simulink library "bcm"  (R2021b)
settings: Solver=VariableStepAuto  StartTime=0.0  StopTime=10.0  RelTol=1e-3
undefined symbols (not defined in the file or in its folder): KBCM_BSDFlashOFFT_cnt, KBCM_BSDFlashONT_cnt, KBCM_BSDRedMode_enum, KBCM_BSDWarnReqLv_enum, KBCM_FireBuzzerEN_flg, KBCM_FLTurnLPLv_A, KBCM_FRTurnLPLv_A, KBCM_LampOFFV_V, KBCM_LampONV_V, KBCM_LightDelayOFFT_Cnt, KBCM_LightDelayONT_Cnt, KBCM_RLTurnLPLv_A, KBCM_RRTurnLPLv_A
libraries: simulink x103, hdlsllib x1
(part 2 of 3)

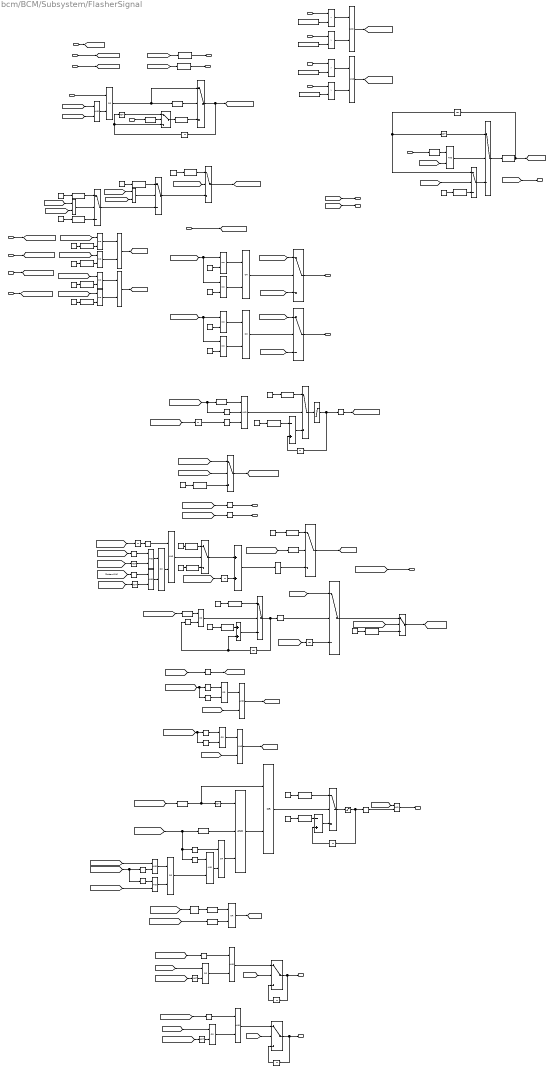
== system bcm/BCM/Subsystem/FlasherSignal ==
  IG1 : Inport
  VINP_LTurnSW_flg : Inport  Port=2
  VINP_RTurnSW_flg : Inport  Port=3
  VINP_VCUHVILSta_flg : Inport  Port=4
  VINP_HazardSW_flg : Inport  Port=5
  VINP_LBSDWarnLv_enum : Inport  Port=6
  VINP_RBSDWarnLv_enum : Inport  Port=7
  VINP_LeftWarnMode_enum : Inport  Port=8
  VINP_RightWarnMode_enum : Inport  Port=9
  PLamp : Inport  Port=10
  VINP_ZFRBCMLFTurnLpCSta_A : Inport  Port=11
  VINP_ZRRBCMLRTurnLpCSta_A : Inport  Port=12
  VINP_ZFRBCMRFTurnLpCSta_A : Inport  Port=13
  VINP_ZRRBCMRRTurnLpCSta_A : Inport  Port=14
  VINP_IVIBuzzerMuteSWSta_flg : Inport  Port=15
  Add : Sum  Inputs=-+
  Add1 : Sum
  Add2 : Sum
  Add3 : Sum  Inputs=-+
  Bit Shift : hdlsllib/Logic and Bit Operations/Bit Shift  mode=Shift Right Logical  N=1
  Bitwise AND : simulink/Logic and Bit Operations/Bitwise Operator  logicop=AND  UseBitMask=on  BitMask=bin2dec('00000011')  BitMaskRealWorld=Stored Integer
  Compare To Constant : simulink/Logic and Bit Operations/Compare To Constant  relop=>  const=0  OutDataTypeStr=boolean
  Compare To Constant1 : simulink/Logic and Bit Operations/Compare To Constant  relop=>  const=0  OutDataTypeStr=boolean
  Compare To Constant10 : simulink/Logic and Bit Operations/Compare To Constant  relop=<  const=2  OutDataTypeStr=boolean
  Compare To Constant11 : simulink/Logic and Bit Operations/Compare To Constant  relop===  const=1  OutDataTypeStr=boolean
  Compare To Constant{3,8,12,17,21} (5 alike) : simulink/Logic and Bit Operations/Compare To Constant  relop===  const=2  OutDataTypeStr=boolean
  Compare To Constant13 : simulink/Logic and Bit Operations/Compare To Constant  relop===  const=1  OutDataTypeStr=boolean
  Compare To Constant{4,9,14,18,23} (5 alike) : simulink/Logic and Bit Operations/Compare To Constant  relop===  const=3  OutDataTypeStr=boolean
  Compare To Constant15 : simulink/Logic and Bit Operations/Compare To Constant  relop===  const=0  OutDataTypeStr=boolean
  Compare To Constant16 : simulink/Logic and Bit Operations/Compare To Constant  relop===  const=1  OutDataTypeStr=boolean
  Compare To Constant19 : simulink/Logic and Bit Operations/Compare To Constant  relop=>  const=0  OutDataTypeStr=boolean
  Compare To Constant2 : simulink/Logic and Bit Operations/Compare To Constant  relop===  const=0  OutDataTypeStr=boolean
  Compare To Constant5 : simulink/Logic and Bit Operations/Compare To Constant  relop=>=  const=17  OutDataTypeStr=boolean
  Compare To Constant6 : simulink/Logic and Bit Operations/Compare To Constant  relop=>=  const=17  OutDataTypeStr=boolean
  Compare To Constant7 : simulink/Logic and Bit Operations/Compare To Constant  relop===  const=0  OutDataTypeStr=boolean
  Constant{,8,10,17..18,20,23,26} (8 alike) : Constant
  Constant{1,4,6,9} (4 alike) : Constant  Value=2
  Constant11 : Constant  Value=3
  Constant12 : Constant  Value=KBCM_FLTurnLPLv_A
  Constant13 : Constant  Value=KBCM_RLTurnLPLv_A
  Constant14 : Constant  Value=KBCM_FRTurnLPLv_A
  Constant15 : Constant  Value=KBCM_RRTurnLPLv_A
  Constant16 : Constant  Value=12
  Constant{3,19,21..22,25} (5 alike) : Constant  Value=0
  Constant2 : Constant  Value=3
  Constant27 : Constant  Value=3
  Constant28 : Constant  Value=10
  Constant5 : Constant  Value=11
  Constant7 : Constant  Value=11
  Data Type Conversion : DataTypeConversion  OutDataTypeStr=boolean
  Data Type Conversion{1..8,12..15,17..19} (15 alike) : DataTypeConversion  OutDataTypeStr=uint8
  Data Type Conversion{9..11,20} (4 alike) : DataTypeConversion  OutDataTypeStr=int8
  Data Type Conversion16 : DataTypeConversion  OutDataTypeStr=boolean
  Data Type Conversion21 : DataTypeConversion  OutDataTypeStr=boolean
  Data Type Conversion22 : DataTypeConversion
  Data Type Conversion23 : DataTypeConversion
  Detect Change{,1..6} (7 alike) : simulink/Logic and Bit Operations/Detect Change  vinit=0  OutDataTypeStr=boolean
  Detect Increase : simulink/Logic and Bit Operations/Detect Increase  vinit=0.0  OutDataTypeStr=boolean
  Detect Increase1 : simulink/Logic and Bit Operations/Detect Increase  vinit=0.0  OutDataTypeStr=boolean
  Detect Increase2 : simulink/Logic and Bit Operations/Detect Increase  vinit=0.0  OutDataTypeStr=boolean
  Logical Operator{,3..6,9..10,17..19,23,25..26,29..30,33,35..36,38} (19 alike) : Logic  AllPortsSameDT=off  OutDataTypeStr=boolean
  Logical Operator{1,13..15,37,39..40} (7 alike) : Logic  Operator=NOT  AllPortsSameDT=off  OutDataTypeStr=boolean
  Logical Operator11 : Logic  Inputs=3  AllPortsSameDT=off  OutDataTypeStr=boolean
  Logical Operator{2,7..8,12,20..22,24,27..28,31..32,34} (13 alike) : Logic  Operator=OR  AllPortsSameDT=off  OutDataTypeStr=boolean
  Logical Operator16 : Logic  Inputs=3  AllPortsSameDT=off  OutDataTypeStr=boolean
  Relational Operator{,1..7} (8 alike) : RelationalOperator  Operator===  OutDataTypeStr=boolean  RndMeth=Simplest
  Relational Operator{8..11} (4 alike) : RelationalOperator  Operator=>  OutDataTypeStr=boolean  RndMeth=Simplest
  Saturation : Saturate  UpperLimit=12  LowerLimit=0
  Saturation1 : Saturate  UpperLimit=10  LowerLimit=0
  Switch{,1..18} (19 alike) : Switch  Criteria=u2 > Threshold
  Unit Delay{,1..10} (11 alike) : UnitDelay  SampleTime=-1  HasFrameUpgradeWarning=on
  VBCM_FDCBCMSMKLCmd_flg : Outport
  VBCM_FDCBCMSMKRCmd_flg : Outport  Port=2
  VBCM_FDCBCMDVRSignalLCmd_flg : Outport  Port=3
  VBCM_FDCBCMDVRSignalRCmd_flg : Outport  Port=4
  VBCM_FDCBCMBSDBuzzerCmd_flg : Outport  Port=5
  VBCM_FDCBCMSLTLpCmd_flg : Outport  Port=6
  VBCM_FDCBCMSRTLpCmd_flg : Outport  Port=7
  VBCM_FDCBCMLTurnLpCmd_flg : Outport  Port=8
  VBCM_FDCBCMRTurnLpCmd_flg : Outport  Port=9
  PatternOld : Outport  Port=10
  VBCM_FDCBCMLTurnSWSta_flg : Outport  Port=11
  VBCM_FDCBCMRTurnSWSta_flg : Outport  Port=12
  VBCM_FDCBCMTurnBuzzerENSta_flg : Outport  Port=13
  wires:
  VINP_HazardSW_flg/1 -> Detect Increase/1
  Unit Delay/1 -> Switch/3, Logical Operator1/1
  Switch/1 -> Data Type Conversion/1
  Data Type Conversion/1 -> Switch1/3
  Detect Increase/1 -> Switch/2
  Logical Operator1/1 -> Switch/1
  VINP_LTurnSW_flg/1 -> [VINP_LTurnSW_flg]
  VINP_RTurnSW_flg/1 -> [VINP_RTurnSW_flg]
  [VINP_LTurnSW_flg] -> Logical Operator/1
  [VINP_RTurnSW_flg] -> Logical Operator/2
  Logical Operator2/1 -> Detect Change6/1, Switch1/1
  Switch1/1 -> Unit Delay/1, [HazardSW]
  Logical Operator/1 -> Logical Operator2/2
  VINP_VCUHVILSta_flg/1 -> Logical Operator2/1
  Switch2/1 -> Switch3/3
  Switch3/1 -> Switch4/3
  [HazardSW] -> Switch4/2
  Data Type Conversion1/1 -> Switch4/1
  Constant/1 -> Data Type Conversion1/1
  IG1/1 -> [IG1]
  Logical Operator3/1 -> Switch3/2
  [IG1] -> Logical Operator3/1
  [VINP_LTurnSW_flg] -> Logical Operator3/2
  Constant1/1 -> Data Type Conversion2/1
  Data Type Conversion2/1 -> Switch3/1
  Data Type Conversion3/1 -> Switch2/1
  Constant2/1 -> Data Type Conversion3/1
  [VINP_RTurnSW_flg] -> Logical Operator4/2
  [IG1] -> Logical Operator4/1
  Logical Operator4/1 -> Switch2/2
  Constant3/1 -> Data Type Conversion4/1
  Data Type Conversion4/1 -> Switch2/3
  Switch4/1 -> [PatternNew]
  Constant4/1 -> Data Type Conversion5/1
  Data Type Conversion5/1 -> Relational Operator/2
  Data Type Conversion6/1 -> Relational Operator1/2
  Constant5/1 -> Data Type Conversion6/1
  Relational Operator/1 -> Logical Operator5/1
  Relational Operator1/1 -> Logical Operator5/2
  Logical Operator5/1 -> [LBSD_En]
  Logical Operator6/1 -> [RBSD_En]
  Relational Operator3/1 -> Logical Operator6/2
  Relational Operator2/1 -> Logical Operator6/1
  Constant7/1 -> Data Type Conversion8/1
  Data Type Conversion8/1 -> Relational Operator3/2
  Data Type Conversion7/1 -> Relational Operator2/2
  Constant6/1 -> Data Type Conversion7/1
  [PatternOld] -> Relational Operator5/1, Relational Operator4/1
  Constant8/1 -> Relational Operator4/2
  Constant9/1 -> Relational Operator5/2
  PLamp/1 -> [PLamp]
  Relational Operator4/1 -> Logical Operator7/1
  Relational Operator5/1 -> Logical Operator7/2
  Logical Operator7/1 -> Switch5/2
  [PLamp] -> Switch5/3
  [LTurnLP] -> Switch5/1
  Switch5/1 -> VBCM_FDCBCMSMKLCmd_flg/1
  Switch6/1 -> VBCM_FDCBCMSMKRCmd_flg/1
  [RTurnLP] -> Switch6/1
  [PLamp] -> Switch6/3
  Logical Operator8/1 -> Switch6/2
  Relational Operator7/1 -> Logical Operator8/2
  Relational Operator6/1 -> Logical Operator8/1
  Constant11/1 -> Relational Operator7/2
  Constant10/1 -> Relational Operator6/2
  [PatternOld] -> Relational Operator6/1, Relational Operator7/1
  VINP_ZFRBCMLFTurnLpCSta_A/1 -> Relational Operator8/1
  Constant12/1 -> Relational Operator8/2
  VINP_ZRRBCMLRTurnLpCSta_A/1 -> Relational Operator9/1
  Constant13/1 -> Relational Operator9/2
  VINP_ZFRBCMRFTurnLpCSta_A/1 -> Relational Operator10/1
  Constant14/1 -> Relational Operator10/2
  Constant15/1 -> Relational Operator11/2
  VINP_ZRRBCMRRTurnLpCSta_A/1 -> Relational Operator11/1
  Relational Operator8/1 -> Logical Operator9/1
  Relational Operator9/1 -> Logical Operator9/2
  Logical Operator9/1 -> [LTurnLPOK]
  Relational Operator10/1 -> Logical Operator10/1
  Relational Operator11/1 -> Logical Operator10/2
  Logical Operator10/1 -> [RTurnLPOK]
  [LTurnLP] -> VBCM_FDCBCMLTurnLpCmd_flg/1
  [RTurnLP] -> VBCM_FDCBCMRTurnLpCmd_flg/1
  [PatternOld] -> Detect Change4/1
  Compare To Constant17/1 -> Logical Operator18/2
  Add3/1 -> Switch13/3
  [LampON] -> Logical Operator28/1
  [RBSD_En] -> Logical Operator40/1
  [LBSD_En] -> Logical Operator39/1
  Saturation1/1 -> Compare To Constant19/1, Unit Delay7/1
  [LTurnLPOK] -> Logical Operator13/1
  [STurnUpdate] -> Switch15/2
  Detect Change4/1 -> Logical Operator24/2
  Bit Shift/1 -> Detect Change5/1
  [Step] -> Bit Shift/1
  Compare To Constant15/1 -> Logical Operator21/1
  [PatternOld] -> Detect Increase1/1
  [LampON] -> Logical Operator27/1
  Switch16/1 -> Unit Delay9/1, VBCM_FDCBCMSRTLpCmd_flg/1
  [LBSD_En] -> Logical Operator18/1
  [PatternOld] -> Compare To Constant18/1, Compare To Constant17/1
  Logical Operator16/1 -> Logical Operator22/2
  Switch10/1 -> Switch14/1
  Compare To Constant19/1 -> Logical Operator38/2
  Compare To Constant23/1 -> Logical Operator26/1
  Add2/1 -> Bitwise AND/1
  [Step] -> Unit Delay6/1
  Unit Delay8/1 -> Switch15/3
  Logical Operator24/1 -> [STurnUpdate]
  Detect Change3/1 -> Logical Operator16/2
  Constant18/1 -> Data Type Conversion11/1
  Detect Change5/1 -> Logical Operator24/1
  Switch13/1 -> Saturation1/1
  Logical Operator20/1 -> Logical Operator17/2
  Detect Increase1/1 -> Logical Operator22/1, Logical Operator15/1
  Logical Operator15/1 -> Logical Operator16/1
  Compare To Constant18/1 -> Logical Operator19/1
  Logical Operator22/1 -> Switch13/2
  Unit Delay9/1 -> Switch16/3
  [RBSD_En] -> Logical Operator19/2
  Logical Operator27/1 -> Logical Operator25/2
  [PatternOld] -> Compare To Constant21/1
  [PatternOld] -> Compare To Constant23/1
  [PatternOld] -> Switch14/2
  Logical Operator25/1 -> Switch15/1
  Constant19/1 -> Data Type Conversion12/1
  Switch12/1 -> Add2/1
  Logical Operator19/1 -> Logical Operator20/2
  Switch14/1 -> [Step]
  Compare To Constant11/1 -> Logical Operator32/1
  Logical Operator32/1 -> Logical Operator33/1
  [NextStep] -> Switch10/1
  Logical Operator14/1 -> Logical Operator30/2
  Unit Delay4/1 -> Compare To Constant7/1
  Compare To Constant10/1 -> [LampON]
  [Step] -> Compare To Constant10/1
  Data Type Conversion12/1 -> Switch14/3
  Data Type Conversion11/1 -> Add3/1
  Compare To Constant12/1 -> Logical Operator32/2
  Constant28/1 -> Data Type Conversion20/1
  [RTurnLPOK] -> Logical Operator14/1
  [LampON] -> Logical Operator35/2
  Compare To Constant14/1 -> Logical Operator34/2
  Compare To Constant16/1 -> Logical Operator17/1
  Logical Operator34/1 -> Logical Operator35/1
  Data Type Conversion19/1 -> Switch12/1
  [Step] -> Unit Delay4/1
  Constant27/1 -> Data Type Conversion19/1
  Logical Operator29/1 -> Logical Operator31/1
  [PatternOld] -> Unit Delay2/1
  Data Type Conversion15/1 -> Add1/1
  Constant23/1 -> Data Type Conversion15/1
  [Step] -> Unit Delay5/1
  [Step] -> Detect Change3/1, Compare To Constant15/1, Compare To Constant16/1
  Logical Operator17/1 -> Logical Operator21/2
  Data Type Conversion18/1 -> Switch12/3
  Unit Delay3/1 -> Compare To Constant5/1, Add1/2
  [PatternOld] -> Compare To Constant3/1
  Bitwise AND/1 -> Switch11/3
  Logical Operator31/1 -> Logical Operator23/2
  Logical Operator11/1 -> Switch7/2
  Add/1 -> Switch7/3
  Compare To Constant6/1 -> Switch10/2
  Constant16/1 -> Data Type Conversion9/1
  Add1/1 -> Switch9/3
  [PatternOld] -> Compare To Constant4/1
  Compare To Constant/1 -> Logical Operator11/3
  Detect Change/1 -> Logical Operator11/1
  Logical Operator30/1 -> Logical Operator31/2
  Unit Delay1/1 -> Add/2
  Logical Operator26/1 -> Switch16/1
  Unit Delay5/1 -> Switch10/3
  Compare To Constant5/1 -> Logical Operator12/2
  [SwitchAllow] -> Switch8/2
  [LampON] -> Logical Operator33/2
  [PatternOld] -> Compare To Constant8/1
  [PatternNew] -> Detect Change/1, Compare To Constant1/1
  Constant25/1 -> Data Type Conversion17/1
  Unit Delay7/1 -> Add3/2
  Constant17/1 -> Data Type Conversion10/1
  Logical Operator28/1 -> Logical Operator26/2
  [STurnUpdate] -> Switch16/2
  Compare To Constant8/1 -> Logical Operator29/1
  Compare To Constant7/1 -> Logical Operator23/1
  Constant22/1 -> Data Type Conversion14/1
  Compare To Constant9/1 -> Logical Operator30/1
  Unit Delay2/1 -> Compare To Constant/1
  Data Type Conversion10/1 -> Add/1
  Switch15/1 -> Unit Delay8/1, VBCM_FDCBCMSLTLpCmd_flg/1
  Detect Change1/1 -> Logical Operator12/1
  Compare To Constant21/1 -> Logical Operator25/1
  Data Type Conversion9/1 -> Switch7/1
  Logical Operator12/1 -> Switch9/2
  Switch11/1 -> [NextStep]
  Switch7/1 -> Saturation/1
  [PatternOld] -> Compare To Constant9/1
  Unit Delay6/1 -> Add2/2
  Logical Operator21/1 -> Logical Operator16/3
  Logical Operator18/1 -> Logical Operator20/1
  Data Type Conversion14/1 -> Switch9/1
  Detect Change2/1 -> Switch11/2
  [PatternOld] -> Detect Change1/1
  Data Type Conversion13/1 -> Switch8/3
  Constant21/1 -> Data Type Conversion13/1
  [PatternOld] -> Compare To Constant13/1, Compare To Constant14/1
  Compare To Constant3/1 -> VBCM_FDCBCMDVRSignalLCmd_flg/1
  Constant26/1 -> Data Type Conversion18/1
  Compare To Constant2/1 -> [SwitchAllow]
  [PatternOld] -> Detect Change2/1
  Data Type Conversion20/1 -> Switch13/1
  Compare To Constant4/1 -> VBCM_FDCBCMDVRSignalRCmd_flg/1
  Switch8/1 -> [PatternOld]
  Compare To Constant13/1 -> Logical Operator34/1
  Logical Operator13/1 -> Logical Operator29/2
  [PatternNew] -> Switch8/1
  [PatternOld] -> Compare To Constant12/1, Compare To Constant11/1
  Compare To Constant1/1 -> Logical Operator11/2
  Logical Operator23/1 -> Switch12/2
  Switch9/1 -> Compare To Constant6/1, Unit Delay3/1
  Data Type Conversion17/1 -> Switch11/1
  Saturation/1 -> Unit Delay1/1, Compare To Constant2/1
  Logical Operator33/1 -> [LTurnLP]
  Logical Operator35/1 -> [RTurnLP]
  [PatternOld] -> PatternOld/1
  VINP_LBSDWarnLv_enum/1 -> [VINP_LBSDWarnLv_enum]
  [VINP_LBSDWarnLv_enum] -> Relational Operator/1
  VINP_LeftWarnMode_enum/1 -> [VINP_LeftWarnMode_enum]
  [VINP_LeftWarnMode_enum] -> Relational Operator1/1
  VINP_RBSDWarnLv_enum/1 -> [VINP_RBSDWarnLv_enum]
  [VINP_RBSDWarnLv_enum] -> Relational Operator2/1
  VINP_RightWarnMode_enum/1 -> [VINP_RightWarnMode_enum]
  [VINP_RightWarnMode_enum] -> Relational Operator3/1
  Detect Change6/1 -> Switch1/2
  [VINP_LTurnSW_flg] -> Data Type Conversion22/1
  [VINP_RTurnSW_flg] -> Data Type Conversion23/1
  VINP_IVIBuzzerMuteSWSta_flg/1 -> Detect Increase2/1
  Detect Increase2/1 -> Logical Operator36/1
  [IG1] -> Logical Operator36/2
  Logical Operator36/1 -> Switch17/2
  Logical Operator37/1 -> Switch17/1
  Switch17/1 -> Data Type Conversion16/1
  Data Type Conversion16/1 -> [TurnBuzzerEN], Unit Delay10/1
  Switch18/1 -> Switch17/3
  [IG1] -> Switch18/2
  Data Type Conversion21/1 -> Switch18/3
  Constant20/1 -> Data Type Conversion21/1
  [TurnBuzzerEN] -> VBCM_FDCBCMTurnBuzzerENSta_flg/1
  [TurnBuzzerEN] -> Logical Operator38/1
  Logical Operator38/1 -> VBCM_FDCBCMBSDBuzzerCmd_flg/1
  Logical Operator39/1 -> Logical Operator27/2
  Logical Operator40/1 -> Logical Operator28/2
  Unit Delay10/1 -> Switch18/1, Logical Operator37/1
  Data Type Conversion22/1 -> VBCM_FDCBCMLTurnSWSta_flg/1
  Data Type Conversion23/1 -> VBCM_FDCBCMRTurnSWSta_flg/1

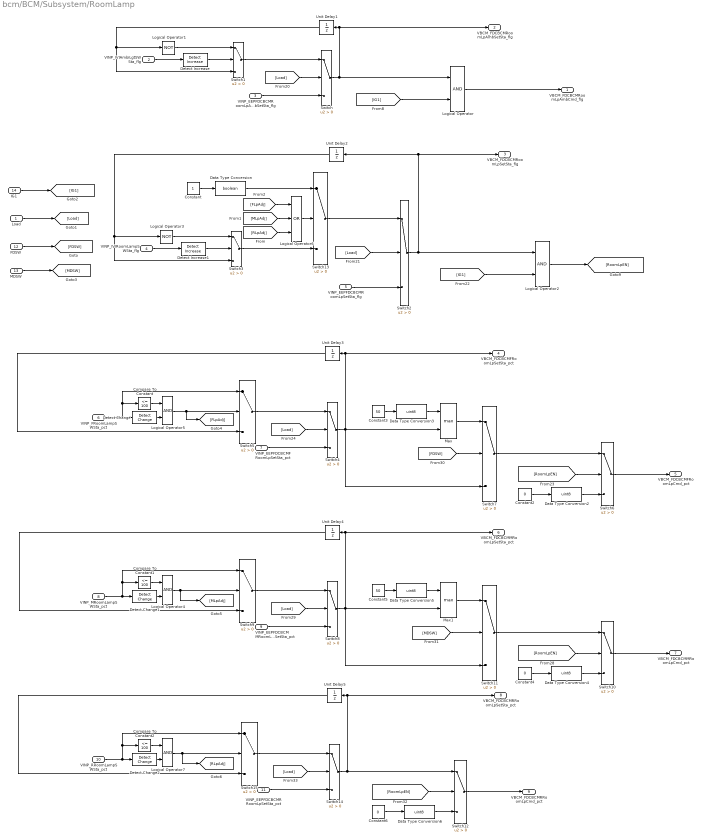
== system bcm/BCM/Subsystem/RoomLamp ==
  Load : Inport
  VINP_IVIAmbiLgtSWSta_flg : Inport  Port=2
  VINP_EEPFDCBCMRoomLpAmbSetSta_flg : Inport  Port=3
  VINP_IVIRoomLampSWSta_flg : Inport  Port=4
  VINP_EEPFDCBCMRoomLpSetSta_flg : Inport  Port=5
  VINP_FRoomLampSWSta_pct : Inport  Port=6
  VINP_EEPFDCBCMFRoomLpSetSta_pct : Inport  Port=7
  VINP_MRoomLampSWSta_pct : Inport  Port=8
  VINP_EEPFDCBCMMRoomLpSetSta_pct : Inport  Port=9
  VINP_RRoomLampSWSta_pct : Inport  Port=10
  VINP_EEPFDCBCMRRoomLpSetSta_pct : Inport  Port=11
  FDSW : Inport  Port=12
  MDSW : Inport  Port=13
  IG1 : Inport  Port=14
  Compare To Constant : simulink/Logic and Bit Operations/Compare To Constant  relop=<=  const=100  OutDataTypeStr=boolean
  Compare To Constant1 : simulink/Logic and Bit Operations/Compare To Constant  relop=<=  const=100  OutDataTypeStr=boolean
  Compare To Constant2 : simulink/Logic and Bit Operations/Compare To Constant  relop=<=  const=100  OutDataTypeStr=boolean
  Constant : Constant
  Constant2 : Constant  Value=0
  Constant3 : Constant  Value=50
  Constant4 : Constant  Value=0
  Constant5 : Constant  Value=50
  Constant6 : Constant  Value=0
  Data Type Conversion : DataTypeConversion  OutDataTypeStr=boolean
  Data Type Conversion{2..6} (5 alike) : DataTypeConversion  OutDataTypeStr=uint8
  Detect Change : simulink/Logic and Bit Operations/Detect Change  vinit=0  OutDataTypeStr=boolean
  Detect Change1 : simulink/Logic and Bit Operations/Detect Change  vinit=0  OutDataTypeStr=boolean
  Detect Change2 : simulink/Logic and Bit Operations/Detect Change  vinit=0  OutDataTypeStr=boolean
  Detect Increase : simulink/Logic and Bit Operations/Detect Increase  vinit=0.0  OutDataTypeStr=boolean
  Detect Increase1 : simulink/Logic and Bit Operations/Detect Increase  vinit=0.0  OutDataTypeStr=boolean
  Logical Operator{,2,4..5,7} (5 alike) : Logic  AllPortsSameDT=off  OutDataTypeStr=boolean
  Logical Operator1 : Logic  Operator=NOT  AllPortsSameDT=off  OutDataTypeStr=boolean
  Logical Operator3 : Logic  Operator=NOT  AllPortsSameDT=off  OutDataTypeStr=boolean
  Logical Operator6 : Logic  Operator=OR  Inputs=3  AllPortsSameDT=off  OutDataTypeStr=boolean
  Max : MinMax  Function=max  Inputs=2
  Max1 : MinMax  Function=max  Inputs=2
  Switch{,1..15} (16 alike) : Switch  Criteria=u2 > Threshold
  Unit Delay{1..5} (5 alike) : UnitDelay  SampleTime=-1  HasFrameUpgradeWarning=on
  VBCM_FDCBCMRoomLpAmbCmd_flg : Outport
  VBCM_FDCBCMRoomLpAmbSetSta_flg : Outport  Port=2
  VBCM_FDCBCMRoomLpSetSta_flg : Outport  Port=3
  VBCM_FDCBCMFRoomLpSetSta_pct : Outport  Port=4
  VBCM_FDCBCMFRoomLpCmd_pct : Outport  Port=5
  VBCM_FDCBCMMRoomLpSetSta_pct : Outport  Port=6
  VBCM_FDCBCMMRoomLpCmd_pct : Outport  Port=7
  VBCM_FDCBCMRRoomLpSetSta_pct : Outport  Port=8
  VBCM_FDCBCMRRoomLpCmd_pct : Outport  Port=9
  wires:
  Data Type Conversion5/1 -> Max1/1
  Logical Operator2/1 -> [RoomLpEN]
  VINP_EEPFDCBCMRRoomLpSetSta_pct/1 -> Switch14/3
  Logical Operator/1 -> VBCM_FDCBCMRoomLpAmbCmd_flg/1
  Compare To Constant/1 -> Logical Operator5/1
  Switch12/1 -> VBCM_FDCBCMRRoomLpCmd_pct/1
  Data Type Conversion2/1 -> Switch6/3
  Switch/1 -> Logical Operator/1, VBCM_FDCBCMRoomLpAmbSetSta_flg/1, Unit Delay1/1
  Logical Operator4/1 -> [MLpAdj], Switch9/2
  VINP_RRoomLampSWSta_pct/1 -> Switch15/1, Compare To Constant2/1, Detect Change2/1
  Switch5/1 -> Switch4/1
  Switch1/1 -> Switch/1
  Switch6/1 -> VBCM_FDCBCMFRoomLpCmd_pct/1
  [FDSW] -> Switch7/2
  Switch14/1 -> Switch12/1, VBCM_FDCBCMRRoomLpSetSta_pct/1, Unit Delay5/1
  [IG1] -> Logical Operator/2
  Switch3/1 -> Switch13/3
  VINP_IVIAmbiLgtSWSta_flg/1 -> Detect Increase/1
  Max1/1 -> Switch11/1
  VINP_IVIRoomLampSWSta_flg/1 -> Detect Increase1/1
  Detect Increase/1 -> Switch1/2
  Unit Delay1/1 -> Logical Operator1/1, Switch1/3
  Data Type Conversion4/1 -> Switch10/3
  [Load] -> Switch2/2
  [MDSW] -> Switch11/2
  Unit Delay2/1 -> Switch3/3, Logical Operator3/1
  Switch2/1 -> Logical Operator2/1, Unit Delay2/1, VBCM_FDCBCMRoomLpSetSta_flg/1
  Logical Operator1/1 -> Switch1/1
  [RoomLpEN] -> Switch6/2
  Logical Operator7/1 -> [RLpAdj], Switch15/2
  VINP_FRoomLampSWSta_pct/1 -> Switch5/1, Compare To Constant/1, Detect Change/1
  Compare To Constant1/1 -> Logical Operator4/1
  Detect Change2/1 -> Logical Operator7/2
  Constant6/1 -> Data Type Conversion6/1
  Constant4/1 -> Data Type Conversion4/1
  [Load] -> Switch/2
  [Load] -> Switch14/2
  Constant3/1 -> Data Type Conversion3/1
  Switch15/1 -> Switch14/1
  VINP_EEPFDCBCMRoomLpAmbSetSta_flg/1 -> Switch/3
  Logical Operator3/1 -> Switch3/1
  Switch7/1 -> Switch6/1
  [IG1] -> Logical Operator2/2
  Switch4/1 -> Switch7/3, VBCM_FDCBCMFRoomLpSetSta_pct/1, Unit Delay3/1, Max/2
  Unit Delay5/1 -> Switch15/3
  Logical Operator5/1 -> [FLpAdj], Switch5/2
  VINP_EEPFDCBCMRoomLpSetSta_flg/1 -> Switch2/3
  Detect Increase1/1 -> Switch3/2
  Data Type Conversion3/1 -> Max/1
  [RoomLpEN] -> Switch12/2
  Data Type Conversion6/1 -> Switch12/3
  Compare To Constant2/1 -> Logical Operator7/1
  [Load] -> Switch4/2
  VINP_EEPFDCBCMFRoomLpSetSta_pct/1 -> Switch4/3
  Unit Delay3/1 -> Switch5/3
  Max/1 -> Switch7/1
  Switch9/1 -> Switch8/1
  Switch11/1 -> Switch10/1
  Constant5/1 -> Data Type Conversion5/1
  Switch10/1 -> VBCM_FDCBCMMRoomLpCmd_pct/1
  Detect Change1/1 -> Logical Operator4/2
  [RoomLpEN] -> Switch10/2
  VINP_MRoomLampSWSta_pct/1 -> Detect Change1/1, Compare To Constant1/1, Switch9/1
  Unit Delay4/1 -> Switch9/3
  Switch8/1 -> Max1/2, VBCM_FDCBCMMRoomLpSetSta_pct/1, Unit Delay4/1, Switch11/3
  Constant2/1 -> Data Type Conversion2/1
  VINP_EEPFDCBCMMRoomLpSetSta_pct/1 -> Switch8/3
  [Load] -> Switch8/2
  Detect Change/1 -> Logical Operator5/2
  FDSW/1 -> [FDSW]
  Load/1 -> [Load]
  IG1/1 -> [IG1]
  MDSW/1 -> [MDSW]
  Switch13/1 -> Switch2/1
  Logical Operator6/1 -> Switch13/2
  [RLpAdj] -> Logical Operator6/3
  [MLpAdj] -> Logical Operator6/2
  [FLpAdj] -> Logical Operator6/1
  Constant/1 -> Data Type Conversion/1
  Data Type Conversion/1 -> Switch13/1

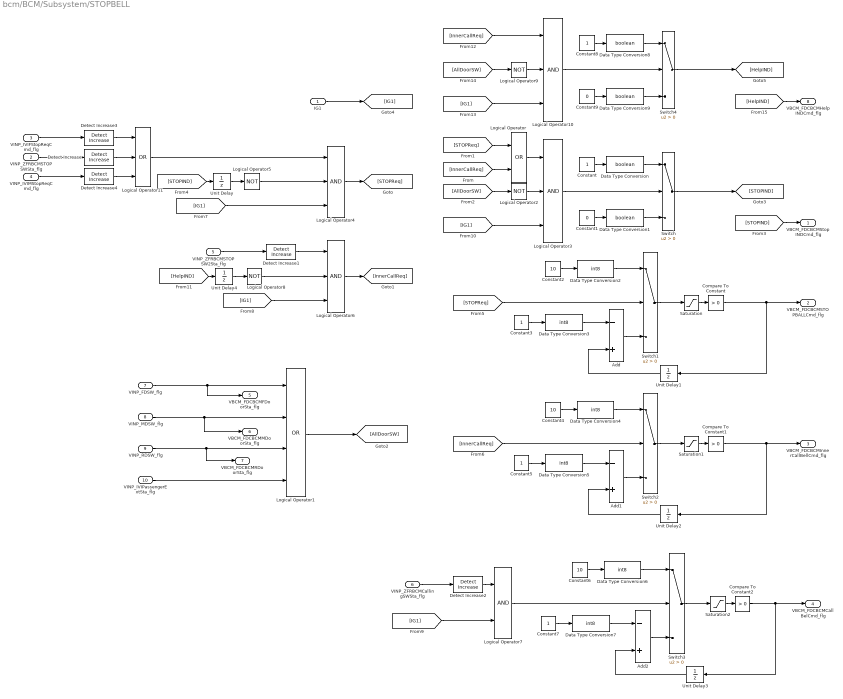
== system bcm/BCM/Subsystem/STOPBELL ==
  IG1 : Inport
  VINP_ZFRBCMSTOPSWSta_flg : Inport  Port=2
  VINP_IVIFStopReqCmd_flg : Inport  Port=3
  VINP_IVIMStopReqCmd_flg : Inport  Port=4
  VINP_ZFRBCMSTOPSW2Sta_flg : Inport  Port=5
  VINP_ZFRBCMCallingSWSta_flg : Inport  Port=6
  VINP_FDSW_flg : Inport  Port=7
  VINP_MDSW_flg : Inport  Port=8
  VINP_RDSW_flg : Inport  Port=9
  VINP_IVIPassengerExtSta_flg : Inport  Port=10
  Add : Sum  Inputs=-+
  Add1 : Sum  Inputs=-+
  Add2 : Sum  Inputs=-+
  Compare To Constant : simulink/Logic and Bit Operations/Compare To Constant  relop=>  const=0  OutDataTypeStr=boolean
  Compare To Constant1 : simulink/Logic and Bit Operations/Compare To Constant  relop=>  const=0  OutDataTypeStr=boolean
  Compare To Constant2 : simulink/Logic and Bit Operations/Compare To Constant  relop=>  const=0  OutDataTypeStr=boolean
  Constant{,3,5,7..8} (5 alike) : Constant
  Constant1 : Constant  Value=0
  Constant2 : Constant  Value=10
  Constant4 : Constant  Value=10
  Constant6 : Constant  Value=10
  Constant9 : Constant  Value=0
  Data Type Conversion{,1,8..9} (4 alike) : DataTypeConversion  OutDataTypeStr=boolean
  Data Type Conversion{2..7} (6 alike) : DataTypeConversion  OutDataTypeStr=int8
  Detect Increase{,1..4} (5 alike) : simulink/Logic and Bit Operations/Detect Increase  vinit=0.0  OutDataTypeStr=boolean
  Logical Operator : Logic  Operator=OR  AllPortsSameDT=off  OutDataTypeStr=boolean
  Logical Operator1 : Logic  Operator=OR  Inputs=4  AllPortsSameDT=off  OutDataTypeStr=boolean
  Logical Operator{3..4,6,10} (4 alike) : Logic  Inputs=3  AllPortsSameDT=off  OutDataTypeStr=boolean
  Logical Operator11 : Logic  Operator=OR  Inputs=3  AllPortsSameDT=off  OutDataTypeStr=boolean
  Logical Operator{2,5,8..9} (4 alike) : Logic  Operator=NOT  AllPortsSameDT=off  OutDataTypeStr=boolean
  Logical Operator7 : Logic  AllPortsSameDT=off  OutDataTypeStr=boolean
  Saturation : Saturate  UpperLimit=10  LowerLimit=0
  Saturation1 : Saturate  UpperLimit=10  LowerLimit=0
  Saturation2 : Saturate  UpperLimit=10  LowerLimit=0
  Switch{,1..4} (5 alike) : Switch  Criteria=u2 > Threshold
  Unit Delay{,1..4} (5 alike) : UnitDelay  SampleTime=-1  HasFrameUpgradeWarning=on
  VBCM_FDCBCMStopINDCmd_flg : Outport
  VBCM_FDCBCMSTOPBALLCmd_flg : Outport  Port=2
  VBCM_FDCBCMInnerCallBellCmd_flg : Outport  Port=3
  VBCM_FDCBCMCallBelCmd_flg : Outport  Port=4
  VBCM_FDCBCMFDoorSta_flg : Outport  Port=5
  VBCM_FDCBCMMDoorSta_flg : Outport  Port=6
  VBCM_FDCBCMRDoorSta_flg : Outport  Port=7
  VBCM_FDCBCMHelpINDCmd_flg : Outport  Port=8
  wires:
  VINP_ZFRBCMSTOPSWSta_flg/1 -> Detect Increase/1
  VINP_ZFRBCMSTOPSW2Sta_flg/1 -> Detect Increase1/1
  [STOPReq] -> Logical Operator/1
  [InnerCallReq] -> Logical Operator/2
  Logical Operator/1 -> Logical Operator3/1
  Constant/1 -> Data Type Conversion/1
  Data Type Conversion/1 -> Switch/1
  VINP_MDSW_flg/1 -> VBCM_FDCBCMMDoorSta_flg/1, Logical Operator1/2
  VINP_FDSW_flg/1 -> VBCM_FDCBCMFDoorSta_flg/1, Logical Operator1/1
  VINP_RDSW_flg/1 -> VBCM_FDCBCMRDoorSta_flg/1, Logical Operator1/3
  Logical Operator1/1 -> [AllDoorSW]
  VINP_IVIPassengerExtSta_flg/1 -> Logical Operator1/4
  [AllDoorSW] -> Logical Operator2/1
  Logical Operator2/1 -> Logical Operator3/2
  Logical Operator3/1 -> Switch/2
  Constant1/1 -> Data Type Conversion1/1
  Data Type Conversion1/1 -> Switch/3
  [STOPIND] -> VBCM_FDCBCMStopINDCmd_flg/1
  Switch/1 -> [STOPIND]
  [STOPIND] -> Unit Delay/1
  VINP_ZFRBCMCallingSWSta_flg/1 -> Detect Increase2/1
  Detect Increase/1 -> Logical Operator11/2
  Unit Delay/1 -> Logical Operator5/1
  Logical Operator4/1 -> [STOPReq]
  Logical Operator5/1 -> Logical Operator4/2
  [STOPReq] -> Switch1/2
  Constant2/1 -> Data Type Conversion2/1
  Data Type Conversion2/1 -> Switch1/1
  Add/1 -> Switch1/3
  Data Type Conversion3/1 -> Add/1
  Constant3/1 -> Data Type Conversion3/1
  Switch1/1 -> Saturation/1
  Saturation/1 -> Compare To Constant/1
  Unit Delay1/1 -> Add/2
  Compare To Constant/1 -> VBCM_FDCBCMSTOPBALLCmd_flg/1, Unit Delay1/1
  Compare To Constant1/1 -> VBCM_FDCBCMInnerCallBellCmd_flg/1, Unit Delay2/1
  Unit Delay2/1 -> Add1/2
  Saturation1/1 -> Compare To Constant1/1
  Switch2/1 -> Saturation1/1
  Constant5/1 -> Data Type Conversion5/1
  Data Type Conversion5/1 -> Add1/1
  Add1/1 -> Switch2/3
  Data Type Conversion4/1 -> Switch2/1
  Constant4/1 -> Data Type Conversion4/1
  [InnerCallReq] -> Switch2/2
  Logical Operator7/1 -> Switch3/2
  Constant6/1 -> Data Type Conversion6/1
  Data Type Conversion6/1 -> Switch3/1
  Add2/1 -> Switch3/3
  Data Type Conversion7/1 -> Add2/1
  Constant7/1 -> Data Type Conversion7/1
  Switch3/1 -> Saturation2/1
  Saturation2/1 -> Compare To Constant2/1
  Unit Delay3/1 -> Add2/2
  Compare To Constant2/1 -> Unit Delay3/1, VBCM_FDCBCMCallBelCmd_flg/1
  IG1/1 -> [IG1]
  [IG1] -> Logical Operator4/3
  Logical Operator6/1 -> [InnerCallReq]
  Detect Increase1/1 -> Logical Operator6/1
  [IG1] -> Logical Operator6/3
  [IG1] -> Logical Operator7/2
  Detect Increase2/1 -> Logical Operator7/1
  [IG1] -> Logical Operator3/3
  [IG1] -> Logical Operator10/3
  Switch4/1 -> [HelpIND]
  [HelpIND] -> VBCM_FDCBCMHelpINDCmd_flg/1
  Data Type Conversion9/1 -> Switch4/3
  Constant9/1 -> Data Type Conversion9/1
  Logical Operator10/1 -> Switch4/2
  Logical Operator9/1 -> Logical Operator10/2
  [AllDoorSW] -> Logical Operator9/1
  Data Type Conversion8/1 -> Switch4/1
  Constant8/1 -> Data Type Conversion8/1
  [InnerCallReq] -> Logical Operator10/1
  Logical Operator8/1 -> Logical Operator6/2
  Unit Delay4/1 -> Logical Operator8/1
  [HelpIND] -> Unit Delay4/1
  VINP_IVIFStopReqCmd_flg/1 -> Detect Increase3/1
  Detect Increase3/1 -> Logical Operator11/1
  Logical Operator11/1 -> Logical Operator4/1
  VINP_IVIMStopReqCmd_flg/1 -> Detect Increase4/1
  Detect Increase4/1 -> Logical Operator11/3

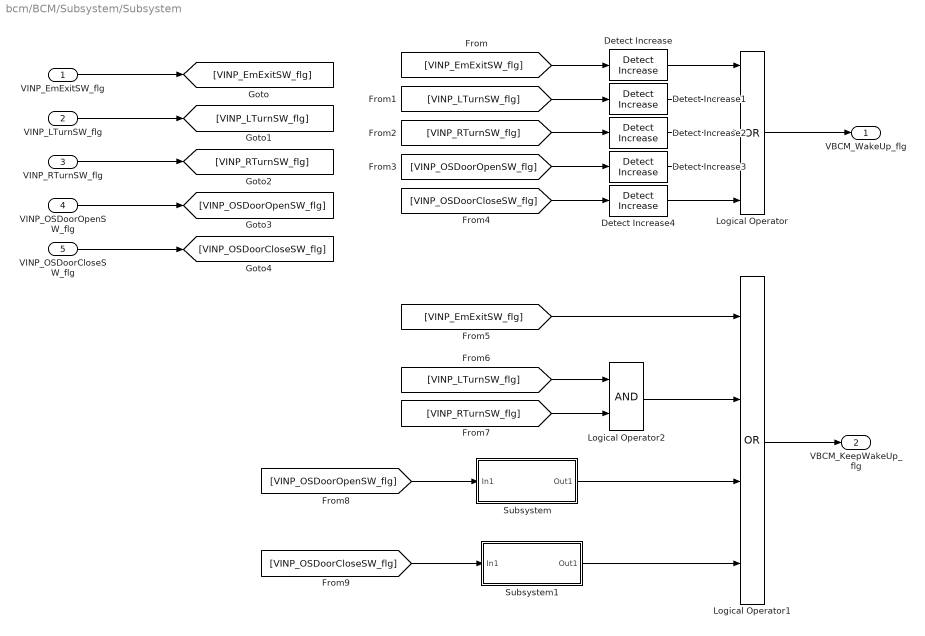
== system bcm/BCM/Subsystem/Subsystem ==
  VINP_EmExitSW_flg : Inport
  VINP_LTurnSW_flg : Inport  Port=2
  VINP_RTurnSW_flg : Inport  Port=3
  VINP_OSDoorOpenSW_flg : Inport  Port=4
  VINP_OSDoorCloseSW_flg : Inport  Port=5
  Detect Increase{,1..4} (5 alike) : simulink/Logic and Bit Operations/Detect Increase  vinit=0.0  OutDataTypeStr=boolean
  Logical Operator : Logic  Operator=OR  Inputs=5  AllPortsSameDT=off  OutDataTypeStr=boolean
  Logical Operator1 : Logic  Operator=OR  Inputs=4  AllPortsSameDT=off  OutDataTypeStr=boolean
  Logical Operator2 : Logic  AllPortsSameDT=off  OutDataTypeStr=boolean
  Subsystem : Subsystem
  Subsystem1 : Subsystem
  VBCM_WakeUp_flg : Outport
  VBCM_KeepWakeUp_flg : Outport  Port=2
  wires:
  VINP_EmExitSW_flg/1 -> [VINP_EmExitSW_flg]
  VINP_LTurnSW_flg/1 -> [VINP_LTurnSW_flg]
  VINP_RTurnSW_flg/1 -> [VINP_RTurnSW_flg]
  VINP_OSDoorOpenSW_flg/1 -> [VINP_OSDoorOpenSW_flg]
  VINP_OSDoorCloseSW_flg/1 -> [VINP_OSDoorCloseSW_flg]
  [VINP_EmExitSW_flg] -> Detect Increase/1
  [VINP_LTurnSW_flg] -> Detect Increase1/1
  [VINP_RTurnSW_flg] -> Detect Increase2/1
  [VINP_OSDoorOpenSW_flg] -> Detect Increase3/1
  [VINP_OSDoorCloseSW_flg] -> Detect Increase4/1
  Detect Increase/1 -> Logical Operator/1
  Detect Increase1/1 -> Logical Operator/2
  Detect Increase2/1 -> Logical Operator/3
  Detect Increase3/1 -> Logical Operator/4
  Detect Increase4/1 -> Logical Operator/5
  Logical Operator/1 -> VBCM_WakeUp_flg/1
  [VINP_EmExitSW_flg] -> Logical Operator1/1
  [VINP_LTurnSW_flg] -> Logical Operator2/1
  [VINP_RTurnSW_flg] -> Logical Operator2/2
  Logical Operator2/1 -> Logical Operator1/2
  [VINP_OSDoorOpenSW_flg] -> Subsystem/1(In1)
  Subsystem/1(Out1) -> Logical Operator1/3
  Subsystem1/1(Out1) -> Logical Operator1/4
  [VINP_OSDoorCloseSW_flg] -> Subsystem1/1(In1)
  Logical Operator1/1 -> VBCM_KeepWakeUp_flg/1

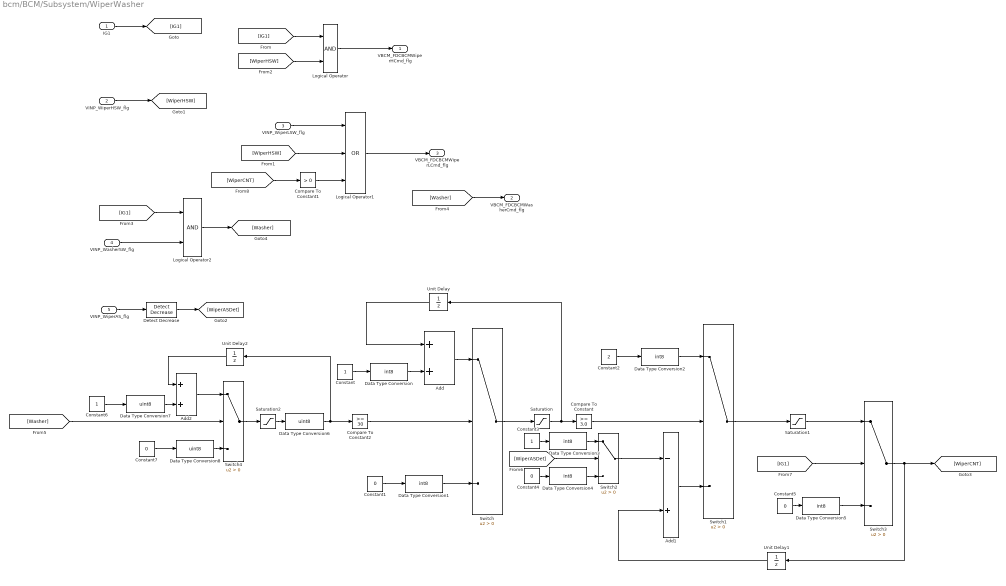
== system bcm/BCM/Subsystem/WiperWasher ==
  IG1 : Inport
  VINP_WiperHSW_flg : Inport  Port=2
  VINP_WiperLSW_flg : Inport  Port=3
  VINP_WasherSW_flg : Inport  Port=4
  VINP_WiperAS_flg : Inport  Port=5
  Add : Sum
  Add1 : Sum  Inputs=-+
  Add2 : Sum
  Compare To Constant : simulink/Logic and Bit Operations/Compare To Constant  relop=>=  const=3.0  OutDataTypeStr=boolean
  Compare To Constant1 : simulink/Logic and Bit Operations/Compare To Constant  relop=>  const=0  OutDataTypeStr=boolean
  Compare To Constant2 : simulink/Logic and Bit Operations/Compare To Constant  relop=>=  const=30  OutDataTypeStr=boolean
  Constant : Constant
  Constant{1,4..5,7} (4 alike) : Constant  Value=0
  Constant2 : Constant  Value=2
  Constant3 : Constant
  Constant6 : Constant
  Data Type Conversion{,1..5} (6 alike) : DataTypeConversion  OutDataTypeStr=int8
  Data Type Conversion6 : DataTypeConversion  OutDataTypeStr=uint8
  Data Type Conversion7 : DataTypeConversion  OutDataTypeStr=uint8
  Data Type Conversion8 : DataTypeConversion  OutDataTypeStr=uint8
  Detect Decrease : simulink/Logic and Bit Operations/Detect Decrease  vinit=0.0  OutDataTypeStr=boolean
  Logical Operator : Logic  AllPortsSameDT=off  OutDataTypeStr=boolean
  Logical Operator1 : Logic  Operator=OR  Inputs=3  AllPortsSameDT=off  OutDataTypeStr=boolean
  Logical Operator2 : Logic  AllPortsSameDT=off  OutDataTypeStr=boolean
  Saturation : Saturate  UpperLimit=3  LowerLimit=0
  Saturation1 : Saturate  UpperLimit=3  LowerLimit=0
  Saturation2 : Saturate  UpperLimit=30  LowerLimit=0
  Switch{,1..4} (5 alike) : Switch  Criteria=u2 > Threshold
  Unit Delay : UnitDelay  SampleTime=-1  HasFrameUpgradeWarning=on
  Unit Delay1 : UnitDelay  SampleTime=-1  HasFrameUpgradeWarning=on
  Unit Delay2 : UnitDelay  SampleTime=-1  HasFrameUpgradeWarning=on
  VBCM_FDCBCMWiperHCmd_flg : Outport
  VBCM_FDCBCMWasherCmd_flg : Outport  Port=2
  VBCM_FDCBCMWiperLCmd_flg : Outport  Port=3
  wires:
  IG1/1 -> [IG1]
  VINP_WiperHSW_flg/1 -> [WiperHSW]
  [IG1] -> Logical Operator/1
  [WiperHSW] -> Logical Operator/2
  Logical Operator/1 -> VBCM_FDCBCMWiperHCmd_flg/1
  VINP_WiperLSW_flg/1 -> Logical Operator1/1
  [WiperHSW] -> Logical Operator1/2
  VINP_WiperAS_flg/1 -> Detect Decrease/1
  Detect Decrease/1 -> [WiperASDet]
  [IG1] -> Logical Operator2/1
  VINP_WasherSW_flg/1 -> Logical Operator2/2
  Logical Operator2/1 -> [Washer]
  [Washer] -> VBCM_FDCBCMWasherCmd_flg/1
  Constant/1 -> Data Type Conversion/1
  Constant1/1 -> Data Type Conversion1/1
  Data Type Conversion/1 -> Add/2
  Add/1 -> Switch/1
  Unit Delay/1 -> Add/1
  Switch/1 -> Saturation/1
  Saturation/1 -> Compare To Constant/1, Unit Delay/1
  Data Type Conversion1/1 -> Switch/3
  Compare To Constant/1 -> Switch1/2
  Constant2/1 -> Data Type Conversion2/1
  Data Type Conversion2/1 -> Switch1/1
  [WiperASDet] -> Switch2/2
  Switch1/1 -> Saturation1/1
  [IG1] -> Switch3/2
  Constant3/1 -> Data Type Conversion3/1
  Data Type Conversion3/1 -> Switch2/1
  Constant4/1 -> Data Type Conversion4/1
  Data Type Conversion4/1 -> Switch2/3
  Switch2/1 -> Add1/1
  Add1/1 -> Switch1/3
  Data Type Conversion5/1 -> Switch3/3
  Constant5/1 -> Data Type Conversion5/1
  Saturation1/1 -> Switch3/1
  Unit Delay1/1 -> Add1/2
  Switch3/1 -> Unit Delay1/1, [WiperCNT]
  [WiperCNT] -> Compare To Constant1/1
  Logical Operator1/1 -> VBCM_FDCBCMWiperLCmd_flg/1
  Compare To Constant1/1 -> Logical Operator1/3
  [Washer] -> Switch4/2
  Add2/1 -> Switch4/1
  Unit Delay2/1 -> Add2/1
  Saturation2/1 -> Data Type Conversion6/1
  Switch4/1 -> Saturation2/1
  Data Type Conversion6/1 -> Compare To Constant2/1, Unit Delay2/1
  Data Type Conversion7/1 -> Add2/2
  Constant6/1 -> Data Type Conversion7/1
  Compare To Constant2/1 -> Switch/2
  Constant7/1 -> Data Type Conversion8/1
  Data Type Conversion8/1 -> Switch4/3

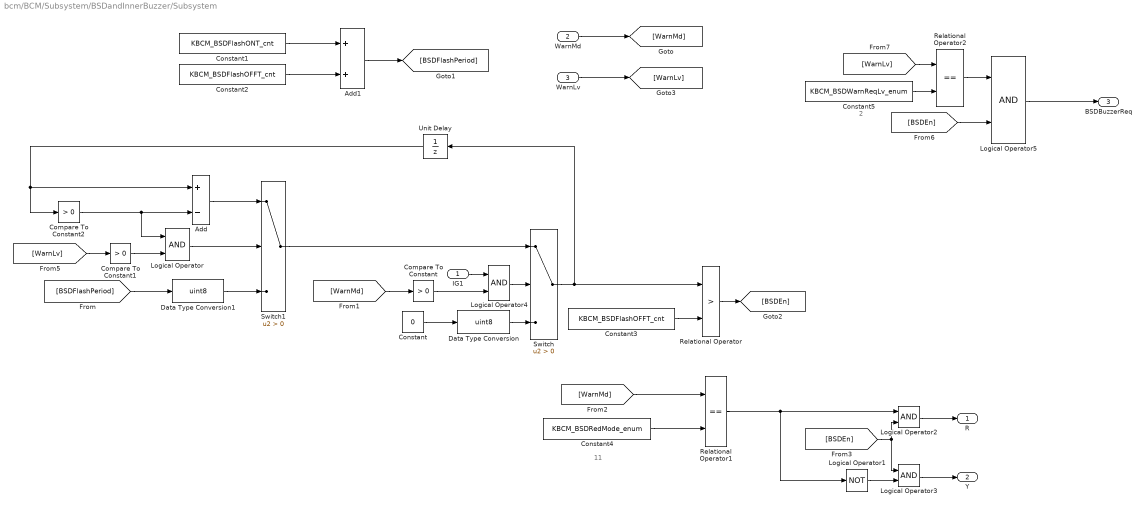
== system bcm/BCM/Subsystem/BSDandInnerBuzzer/Subsystem ==
  note: 2
  note: 11
  IG1 : Inport
  WarnMd : Inport  Port=2
  WarnLv : Inport  Port=3
  Add : Sum  Inputs=+-
  Add1 : Sum
  Compare To Constant : simulink/Logic and Bit Operations/Compare To Constant  relop=>  const=0  OutDataTypeStr=boolean
  Compare To Constant1 : simulink/Logic and Bit Operations/Compare To Constant  relop=>  const=0  OutDataTypeStr=boolean
  Compare To Constant2 : simulink/Logic and Bit Operations/Compare To Constant  relop=>  const=0  OutDataTypeStr=boolean
  Constant : Constant  Value=0
  Constant1 : Constant  Value=KBCM_BSDFlashONT_cnt
  Constant2 : Constant  Value=KBCM_BSDFlashOFFT_cnt
  Constant3 : Constant  Value=KBCM_BSDFlashOFFT_cnt
  Constant4 : Constant  Value=KBCM_BSDRedMode_enum
  Constant5 : Constant  Value=KBCM_BSDWarnReqLv_enum
  Data Type Conversion : DataTypeConversion  OutDataTypeStr=uint8
  Data Type Conversion1 : DataTypeConversion  OutDataTypeStr=uint8
  Logical Operator{,2..5} (5 alike) : Logic  AllPortsSameDT=off  OutDataTypeStr=boolean
  Logical Operator1 : Logic  Operator=NOT  AllPortsSameDT=off  OutDataTypeStr=boolean
  Relational Operator : RelationalOperator  Operator=>  OutDataTypeStr=boolean  RndMeth=Simplest
  Relational Operator1 : RelationalOperator  Operator===  OutDataTypeStr=boolean  RndMeth=Simplest
  Relational Operator2 : RelationalOperator  Operator===  OutDataTypeStr=boolean  RndMeth=Simplest
  Switch : Switch  Criteria=u2 > Threshold
  Switch1 : Switch  Criteria=u2 > Threshold
  Unit Delay : UnitDelay  SampleTime=-1  HasFrameUpgradeWarning=on
  R : Outport
  Y : Outport  Port=2
  BSDBuzzerReq : Outport  Port=3
  wires:
  Compare To Constant/1 -> Logical Operator4/2
  Data Type Conversion/1 -> Switch/3
  Constant/1 -> Data Type Conversion/1
  Compare To Constant1/1 -> Logical Operator/2
  Unit Delay/1 -> Compare To Constant2/1, Add/1
  Add/1 -> Switch1/1
  Compare To Constant2/1 -> Logical Operator/1, Add/2
  Switch1/1 -> Switch/1
  Add1/1 -> [BSDFlashPeriod]
  Constant1/1 -> Add1/1
  Constant2/1 -> Add1/2
  Data Type Conversion1/1 -> Switch1/3
  [BSDFlashPeriod] -> Data Type Conversion1/1
  Logical Operator/1 -> Switch1/2
  Switch/1 -> Relational Operator/1, Unit Delay/1
  Constant3/1 -> Relational Operator/2
  WarnMd/1 -> [WarnMd]
  [WarnMd] -> Compare To Constant/1
  Relational Operator/1 -> [BSDEn]
  [BSDEn] -> Logical Operator3/1, Logical Operator2/2
  Constant4/1 -> Relational Operator1/2
  Relational Operator1/1 -> Logical Operator1/1, Logical Operator2/1
  Logical Operator1/1 -> Logical Operator3/2
  Logical Operator2/1 -> R/1
  Logical Operator3/1 -> Y/1
  Logical Operator4/1 -> Switch/2
  IG1/1 -> Logical Operator4/1
  WarnLv/1 -> [WarnLv]
  [WarnLv] -> Compare To Constant1/1
  [WarnLv] -> Relational Operator2/1
  Constant5/1 -> Relational Operator2/2
  Relational Operator2/1 -> Logical Operator5/1
  [BSDEn] -> Logical Operator5/2
  Logical Operator5/1 -> BSDBuzzerReq/1
  [WarnMd] -> Relational Operator1/1

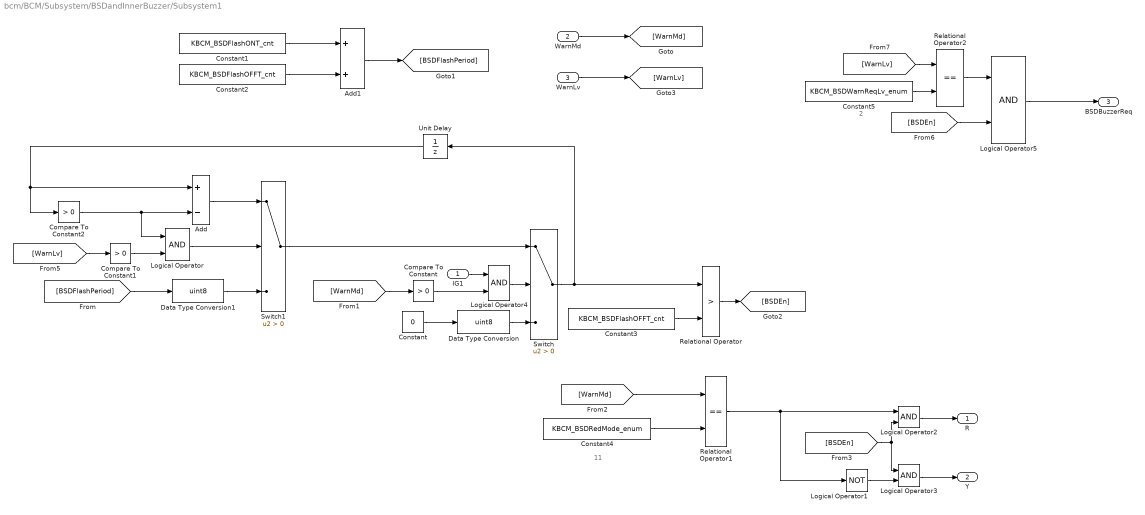
== system bcm/BCM/Subsystem/BSDandInnerBuzzer/Subsystem1 ==
  note: 11
  note: 2
  IG1 : Inport
  WarnMd : Inport  Port=2
  WarnLv : Inport  Port=3
  Add : Sum  Inputs=+-
  Add1 : Sum
  Compare To Constant : simulink/Logic and Bit Operations/Compare To Constant  relop=>  const=0  OutDataTypeStr=boolean
  Compare To Constant1 : simulink/Logic and Bit Operations/Compare To Constant  relop=>  const=0  OutDataTypeStr=boolean
  Compare To Constant2 : simulink/Logic and Bit Operations/Compare To Constant  relop=>  const=0  OutDataTypeStr=boolean
  Constant : Constant  Value=0
  Constant1 : Constant  Value=KBCM_BSDFlashONT_cnt
  Constant2 : Constant  Value=KBCM_BSDFlashOFFT_cnt
  Constant3 : Constant  Value=KBCM_BSDFlashOFFT_cnt
  Constant4 : Constant  Value=KBCM_BSDRedMode_enum
  Constant5 : Constant  Value=KBCM_BSDWarnReqLv_enum
  Data Type Conversion : DataTypeConversion  OutDataTypeStr=uint8
  Data Type Conversion1 : DataTypeConversion  OutDataTypeStr=uint8
  Logical Operator{,2..5} (5 alike) : Logic  AllPortsSameDT=off  OutDataTypeStr=boolean
  Logical Operator1 : Logic  Operator=NOT  AllPortsSameDT=off  OutDataTypeStr=boolean
  Relational Operator : RelationalOperator  Operator=>  OutDataTypeStr=boolean  RndMeth=Simplest
  Relational Operator1 : RelationalOperator  Operator===  OutDataTypeStr=boolean  RndMeth=Simplest
  Relational Operator2 : RelationalOperator  Operator===  OutDataTypeStr=boolean  RndMeth=Simplest
  Switch : Switch  Criteria=u2 > Threshold
  Switch1 : Switch  Criteria=u2 > Threshold
  Unit Delay : UnitDelay  SampleTime=-1  HasFrameUpgradeWarning=on
  R : Outport
  Y : Outport  Port=2
  BSDBuzzerReq : Outport  Port=3
  wires:
  [WarnMd] -> Relational Operator1/1
  Logical Operator5/1 -> BSDBuzzerReq/1
  [BSDEn] -> Logical Operator5/2
  Relational Operator2/1 -> Logical Operator5/1
  Constant5/1 -> Relational Operator2/2
  [WarnLv] -> Relational Operator2/1
  [WarnLv] -> Compare To Constant1/1
  WarnLv/1 -> [WarnLv]
  IG1/1 -> Logical Operator4/1
  Logical Operator4/1 -> Switch/2
  Logical Operator3/1 -> Y/1
  Logical Operator2/1 -> R/1
  Logical Operator1/1 -> Logical Operator3/2
  Relational Operator1/1 -> Logical Operator2/1, Logical Operator1/1
  Constant4/1 -> Relational Operator1/2
  [BSDEn] -> Logical Operator3/1, Logical Operator2/2
  Relational Operator/1 -> [BSDEn]
  [WarnMd] -> Compare To Constant/1
  WarnMd/1 -> [WarnMd]
  Constant3/1 -> Relational Operator/2
  Switch/1 -> Unit Delay/1, Relational Operator/1
  Logical Operator/1 -> Switch1/2
  [BSDFlashPeriod] -> Data Type Conversion1/1
  Data Type Conversion1/1 -> Switch1/3
  Constant2/1 -> Add1/2
  Constant1/1 -> Add1/1
  Add1/1 -> [BSDFlashPeriod]
  Switch1/1 -> Switch/1
  Compare To Constant2/1 -> Add/2, Logical Operator/1
  Add/1 -> Switch1/1
  Unit Delay/1 -> Add/1, Compare To Constant2/1
  Compare To Constant1/1 -> Logical Operator/2
  Constant/1 -> Data Type Conversion/1
  Data Type Conversion/1 -> Switch/3
  Compare To Constant/1 -> Logical Operator4/2

== system bcm/BCM/Subsystem/DoorControl/Subsystem ==
  IG1 : Inport
  SWin : Inport  Port=2
  Moving : Inport  Port=3
  Add : Sum  Inputs=-+
  Compare To Constant1 : simulink/Logic and Bit Operations/Compare To Constant  relop=>  const=0  OutDataTypeStr=boolean
  Constant : Constant  Value=20
  Constant1 : Constant
  Constant2 : Constant  Value=0
  Data Type Conversion : DataTypeConversion  OutDataTypeStr=uint8
  Data Type Conversion1 : DataTypeConversion  OutDataTypeStr=uint8
  Data Type Conversion2 : DataTypeConversion  OutDataTypeStr=uint8
  Data Type Conversion3 : DataTypeConversion  OutDataTypeStr=boolean
  Detect Increase2 : simulink/Logic and Bit Operations/Detect Increase  vinit=0.0  OutDataTypeStr=boolean
  Logical Operator5 : Logic  Inputs=3  AllPortsSameDT=off  OutDataTypeStr=boolean
  Logical Operator6 : Logic  Operator=NOT  AllPortsSameDT=off  OutDataTypeStr=boolean
  Switch : Switch  Criteria=u2 > Threshold
  Switch1 : Switch  Criteria=u2 > Threshold
  Unit Delay : UnitDelay  SampleTime=-1  HasFrameUpgradeWarning=on
  Cmd : Outport
  wires:
  Data Type Conversion1/1 -> Switch1/1
  Switch1/1 -> Add/1
  Compare To Constant1/1 -> Switch1/2
  Unit Delay/1 -> Add/2, Compare To Constant1/1
  Detect Increase2/1 -> Logical Operator5/2
  Moving/1 -> Logical Operator6/1
  IG1/1 -> Logical Operator5/1
  Switch/1 -> Data Type Conversion3/1
  Data Type Conversion/1 -> Switch/1
  Constant1/1 -> Data Type Conversion1/1
  Data Type Conversion3/1 -> Cmd/1, Unit Delay/1
  Data Type Conversion2/1 -> Switch1/3
  Logical Operator6/1 -> Logical Operator5/3
  Constant/1 -> Data Type Conversion/1
  Constant2/1 -> Data Type Conversion2/1
  Logical Operator5/1 -> Switch/2
  SWin/1 -> Detect Increase2/1
  Add/1 -> Switch/3

== system bcm/BCM/Subsystem/DoorControl/Subsystem1 ==
  IG1 : Inport
  SWin : Inport  Port=2
  Moving : Inport  Port=3
  Add : Sum  Inputs=-+
  Compare To Constant1 : simulink/Logic and Bit Operations/Compare To Constant  relop=>  const=0  OutDataTypeStr=boolean
  Constant : Constant  Value=20
  Constant1 : Constant
  Constant2 : Constant  Value=0
  Data Type Conversion : DataTypeConversion  OutDataTypeStr=uint8
  Data Type Conversion1 : DataTypeConversion  OutDataTypeStr=uint8
  Data Type Conversion2 : DataTypeConversion  OutDataTypeStr=uint8
  Data Type Conversion3 : DataTypeConversion  OutDataTypeStr=boolean
  Detect Increase2 : simulink/Logic and Bit Operations/Detect Increase  vinit=0.0  OutDataTypeStr=boolean
  Logical Operator5 : Logic  Inputs=3  AllPortsSameDT=off  OutDataTypeStr=boolean
  Logical Operator6 : Logic  Operator=NOT  AllPortsSameDT=off  OutDataTypeStr=boolean
  Switch : Switch  Criteria=u2 > Threshold
  Switch1 : Switch  Criteria=u2 > Threshold
  Unit Delay : UnitDelay  SampleTime=-1  HasFrameUpgradeWarning=on
  Cmd : Outport
  wires:
  Add/1 -> Switch/3
  SWin/1 -> Detect Increase2/1
  Logical Operator5/1 -> Switch/2
  Constant2/1 -> Data Type Conversion2/1
  Constant/1 -> Data Type Conversion/1
  Logical Operator6/1 -> Logical Operator5/3
  Data Type Conversion2/1 -> Switch1/3
  Data Type Conversion3/1 -> Unit Delay/1, Cmd/1
  Constant1/1 -> Data Type Conversion1/1
  Data Type Conversion/1 -> Switch/1
  Switch/1 -> Data Type Conversion3/1
  IG1/1 -> Logical Operator5/1
  Moving/1 -> Logical Operator6/1
  Detect Increase2/1 -> Logical Operator5/2
  Unit Delay/1 -> Compare To Constant1/1, Add/2
  Compare To Constant1/1 -> Switch1/2
  Switch1/1 -> Add/1
  Data Type Conversion1/1 -> Switch1/1

== system bcm/BCM/Subsystem/DoorControl/Subsystem2 ==
  IG1 : Inport
  SWin : Inport  Port=2
  Moving : Inport  Port=3
  Add : Sum  Inputs=-+
  Compare To Constant1 : simulink/Logic and Bit Operations/Compare To Constant  relop=>  const=0  OutDataTypeStr=boolean
  Constant : Constant  Value=20
  Constant1 : Constant
  Constant2 : Constant  Value=0
  Data Type Conversion : DataTypeConversion  OutDataTypeStr=uint8
  Data Type Conversion1 : DataTypeConversion  OutDataTypeStr=uint8
  Data Type Conversion2 : DataTypeConversion  OutDataTypeStr=uint8
  Data Type Conversion3 : DataTypeConversion  OutDataTypeStr=boolean
  Detect Increase2 : simulink/Logic and Bit Operations/Detect Increase  vinit=0.0  OutDataTypeStr=boolean
  Logical Operator5 : Logic  Inputs=3  AllPortsSameDT=off  OutDataTypeStr=boolean
  Logical Operator6 : Logic  Operator=NOT  AllPortsSameDT=off  OutDataTypeStr=boolean
  Switch : Switch  Criteria=u2 > Threshold
  Switch1 : Switch  Criteria=u2 > Threshold
  Unit Delay : UnitDelay  SampleTime=-1  HasFrameUpgradeWarning=on
  Cmd : Outport
  wires:
  Data Type Conversion1/1 -> Switch1/1
  Switch1/1 -> Add/1
  Compare To Constant1/1 -> Switch1/2
  Unit Delay/1 -> Add/2, Compare To Constant1/1
  Detect Increase2/1 -> Logical Operator5/2
  Moving/1 -> Logical Operator6/1
  IG1/1 -> Logical Operator5/1
  Switch/1 -> Data Type Conversion3/1
  Data Type Conversion/1 -> Switch/1
  Constant1/1 -> Data Type Conversion1/1
  Data Type Conversion3/1 -> Cmd/1, Unit Delay/1
  Data Type Conversion2/1 -> Switch1/3
  Logical Operator6/1 -> Logical Operator5/3
  Constant/1 -> Data Type Conversion/1
  Constant2/1 -> Data Type Conversion2/1
  Logical Operator5/1 -> Switch/2
  SWin/1 -> Detect Increase2/1
  Add/1 -> Switch/3

== system bcm/BCM/Subsystem/DoorControl/Subsystem3 ==
  IG1 : Inport
  SWin : Inport  Port=2
  Moving : Inport  Port=3
  Add : Sum  Inputs=-+
  Compare To Constant1 : simulink/Logic and Bit Operations/Compare To Constant  relop=>  const=0  OutDataTypeStr=boolean
  Constant : Constant  Value=20
  Constant1 : Constant
  Constant2 : Constant  Value=0
  Data Type Conversion : DataTypeConversion  OutDataTypeStr=uint8
  Data Type Conversion1 : DataTypeConversion  OutDataTypeStr=uint8
  Data Type Conversion2 : DataTypeConversion  OutDataTypeStr=uint8
  Data Type Conversion3 : DataTypeConversion  OutDataTypeStr=boolean
  Detect Increase2 : simulink/Logic and Bit Operations/Detect Increase  vinit=0.0  OutDataTypeStr=boolean
  Logical Operator5 : Logic  Inputs=3  AllPortsSameDT=off  OutDataTypeStr=boolean
  Logical Operator6 : Logic  Operator=NOT  AllPortsSameDT=off  OutDataTypeStr=boolean
  Switch : Switch  Criteria=u2 > Threshold
  Switch1 : Switch  Criteria=u2 > Threshold
  Unit Delay : UnitDelay  SampleTime=-1  HasFrameUpgradeWarning=on
  Cmd : Outport
  wires:
  Add/1 -> Switch/3
  SWin/1 -> Detect Increase2/1
  Logical Operator5/1 -> Switch/2
  Constant2/1 -> Data Type Conversion2/1
  Constant/1 -> Data Type Conversion/1
  Logical Operator6/1 -> Logical Operator5/3
  Data Type Conversion2/1 -> Switch1/3
  Data Type Conversion3/1 -> Unit Delay/1, Cmd/1
  Constant1/1 -> Data Type Conversion1/1
  Data Type Conversion/1 -> Switch/1
  Switch/1 -> Data Type Conversion3/1
  IG1/1 -> Logical Operator5/1
  Moving/1 -> Logical Operator6/1
  Detect Increase2/1 -> Logical Operator5/2
  Unit Delay/1 -> Compare To Constant1/1, Add/2
  Compare To Constant1/1 -> Switch1/2
  Switch1/1 -> Add/1
  Data Type Conversion1/1 -> Switch1/1

== system bcm/BCM/Subsystem/ExteriorLight/Subsystem4 ==
  note: 3
  note: 2.5
  VINP_LightSensorV_V : Inport
  VINP_AutoLightSW_flg : Inport  Port=2
  IG1 : Inport  Port=3
  Constant1 : Constant  Value=KBCM_LampONV_V
  Constant2 : Constant  Value=KBCM_LampOFFV_V
  DelayOFF : Subsystem
  DelayON : Subsystem
  Logical Operator{,2..4} (4 alike) : Logic  AllPortsSameDT=off  OutDataTypeStr=boolean
  Logical Operator1 : Logic  Operator=OR  AllPortsSameDT=off  OutDataTypeStr=boolean
  Relational Operator : RelationalOperator  Operator=>  OutDataTypeStr=boolean  RndMeth=Simplest
  Relational Operator1 : RelationalOperator  Operator=>  OutDataTypeStr=boolean  RndMeth=Simplest
  Unit Delay : UnitDelay  SampleTime=-1  HasFrameUpgradeWarning=on
  LSensorReq : Outport
  wires:
  VINP_LightSensorV_V/1 -> Relational Operator1/1, Relational Operator/1
  Logical Operator4/1 -> LSensorReq/1, Unit Delay/1
  Constant1/1 -> Relational Operator/2
  Constant2/1 -> Relational Operator1/2
  Relational Operator1/1 -> DelayOFF/1(Low)
  Unit Delay/1 -> Logical Operator/2
  Relational Operator/1 -> Logical Operator3/2
  Logical Operator/1 -> Logical Operator1/2
  DelayOFF/1(DelayOFF) -> Logical Operator/1
  DelayON/1(DelayON) -> Logical Operator1/1
  VINP_AutoLightSW_flg/1 -> Logical Operator2/1
  IG1/1 -> Logical Operator2/2
  Logical Operator2/1 -> [AutoFuncEN]
  [AutoFuncEN] -> Logical Operator3/1
  Logical Operator3/1 -> DelayON/1(High)
  Logical Operator1/1 -> Logical Operator4/1
  [AutoFuncEN] -> Logical Operator4/2
